simulink model "W2_PROB2"  (R2020b)
settings: Solver=VariableStepAuto  StartTime=0.0  StopTime=10.0  RelTol=1e-3
settings Model: Creator=ADMIN  LastModifiedBy=ADMIN

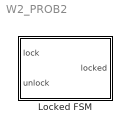
== system W2_PROB2 ==
  Locked FSM : Subsystem

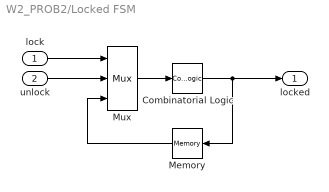
== system W2_PROB2/Locked FSM ==
  lock : Inport
  unlock : Inport  Port=2
  Combinatorial Logic : CombinatorialLogic  TruthTable=[0;1;0;0;1;1;1;0]
  Memory : Memory
  Mux : Mux  Inputs=3
  locked : Outport  InitialOutput=0  VectorParamsAs1DForOutWhenUnconnected=off
  wires:
  lock/1 -> Mux/1
  Memory/1 -> Mux/3
  Combinatorial Logic/1 -> locked/1, Memory/1
  Mux/1 -> Combinatorial Logic/1
  unlock/1 -> Mux/2
